simulink model "SingleTrackCANoe"  (R2021b)
settings: Solver=ode1  StartTime=0  StopTime=2  FixedStep=1.0000000000000000e-003  RelTol=1e-3
InitFcn:
  | sampleTime = str2double(get_param(bdroot, 'FixedStep'));
undefined symbols (not defined in the file or in its folder): AccPedalPos, BrakePedalPos, BrakeSwitch, DiscIntNeverNeededParam, DYNA4, EngSpd, IgnitionSwitch, InitialGear, InitialSpeed, IntendedEngTrq, LeftIndicator, MainBrakePress, MaxGear, MDL, MinGear, RefAcc, RefLane, RefLatPos, RefPath, RefPathCurv, RefSpd, RefSpdPreview, RefSpdRetrospect, RightIndicator, SteeringWheelAng, SteeringWheelTrq, UserDefinedRefValue, vm_const
libraries: UtilitiesLibrary x62, simulink x18, WheelSystemModules x14, LongitudinalControllerModules x13, LateralControllerModules x7, AnimationBusselectorModules x5, EnvironmentModules x5, BasicEngineControlModules x5, MiscellaneousControlModules x5, Animation3Modules x4, AuxiliariesModules x4, ReducedTireModules x4
(part 19 of 34)

== system SingleTrackCANoe/SimulationModel/Vehicle/Drivetrain/DrivetrainControlUnit/InputFromCTRL ==
  fromCTRL : Inport
  TDBusSelector : BusSelector  OutputSignals=CTRL.LongitudinalControl.TransmissionLoad[0_1],CTRL.LongitudinalControl.IntendedEngTrqActive[0;1],CTRL.LongitudinalControl.AccPedalPos[0_1],CTRL.LongitudinalControl.InitialGear[-4;20],CTRL.LongitudinalControl.MaxGear[-4;20],CTRL.LongitudinalControl.MinGear[-4;20],CTRL.LongitudinalControl.ShiftingProgramSelection[-],CTRL.LongitudinalControl.KickdownSwitch[0;1]
  __TDD__AccPedalPos[0_1] : Demux  Outputs=[1]
  __TDD__InitialGear[-4;20] : Demux  Outputs=[1]
  __TDD__IntendedEngTrqActive[0;1] : Demux  Outputs=[1]
  __TDD__KickdownSwitch[0;1] : Demux  Outputs=[1]
  __TDD__MaxGear[-4;20] : Demux  Outputs=[1]
  __TDD__MinGear[-4;20] : Demux  Outputs=[1]
  __TDD__ShiftingProgramSelection[-] : Demux  Outputs=[1]
  __TDD__TransmissionLoad[0_1] : Demux  Outputs=[1]
  TransmissionLoad[0_1]___UNIQUE_1 : Outport  Description=|  PortDimensions=[1]  VectorParamsAs1DForOutWhenUnconnected=off
      | <name>CTRL.LongitudinalControl.TransmissionLoad[0_1]</name>
      | <comment></comment>
  IntendedEngTrqActive[0;1]___UNIQUE_1 : Outport  Description=|  Port=2  PortDimensions=[1]  VectorParamsAs1DForOutWhenUnconnected=off
      | <name>CTRL.LongitudinalControl.IntendedEngTrqActive[0;1]</name>
      | <comment></comment>
  AccPedalPos[0_1]___UNIQUE_1 : Outport  Description=|  Port=3  PortDimensions=[1]  VectorParamsAs1DForOutWhenUnconnected=off
      | <name>CTRL.LongitudinalControl.AccPedalPos[0_1]</name>
      | <comment></comment>
  InitialGear[-4;20]___UNIQUE_1 : Outport  Description=|  Port=4  PortDimensions=[1]  VectorParamsAs1DForOutWhenUnconnected=off
      | <name>CTRL.LongitudinalControl.InitialGear[-4;20]</name>
      | <comment></comment>
  MaxGear[-4;20]___UNIQUE_1 : Outport  Description=|  Port=5  PortDimensions=[1]  VectorParamsAs1DForOutWhenUnconnected=off
      | <name>CTRL.LongitudinalControl.MaxGear[-4;20]</name>
      | <comment>Maximum gear</comment>
  MinGear[-4;20]___UNIQUE_1 : Outport  Description=|  Port=6  PortDimensions=[1]  VectorParamsAs1DForOutWhenUnconnected=off
      | <name>CTRL.LongitudinalControl.MinGear[-4;20]</name>
      | <comment>Minimum gear</comment>
  ShiftingProgramSelection[-]___UNIQUE_1 : Outport  Description=|  Port=7  PortDimensions=[1]  VectorParamsAs1DForOutWhenUnconnected=off
      | <name>CTRL.LongitudinalControl.ShiftingProgramSelection[-]</name>
      | <comment>Shifting program selection</comment>
  KickdownSwitch[0;1]___UNIQUE_1 : Outport  Description=|  Port=8  PortDimensions=[1]  VectorParamsAs1DForOutWhenUnconnected=off
      | <name>CTRL.LongitudinalControl.KickdownSwitch[0;1]</name>
      | <comment>Kickdown switch</comment>
  wires:
  __TDD__KickdownSwitch[0;1]/1 -> KickdownSwitch[0;1]___UNIQUE_1/1  "KickdownSwitch[0;1]"
  __TDD__ShiftingProgramSelection[-]/1 -> ShiftingProgramSelection[-]___UNIQUE_1/1  "ShiftingProgramSelection[-]"
  __TDD__MinGear[-4;20]/1 -> MinGear[-4;20]___UNIQUE_1/1  "MinGear[-4;20]"
  __TDD__MaxGear[-4;20]/1 -> MaxGear[-4;20]___UNIQUE_1/1  "MaxGear[-4;20]"
  __TDD__InitialGear[-4;20]/1 -> InitialGear[-4;20]___UNIQUE_1/1  "InitialGear[-4;20]"
  __TDD__AccPedalPos[0_1]/1 -> AccPedalPos[0_1]___UNIQUE_1/1  "AccPedalPos[0_1]"
  __TDD__IntendedEngTrqActive[0;1]/1 -> IntendedEngTrqActive[0;1]___UNIQUE_1/1  "IntendedEngTrqActive[0;1]"
  __TDD__TransmissionLoad[0_1]/1 -> TransmissionLoad[0_1]___UNIQUE_1/1  "TransmissionLoad[0_1]"
  TDBusSelector/8 -> __TDD__KickdownSwitch[0;1]/1  "<KickdownSwitch[0;1]>"
  TDBusSelector/7 -> __TDD__ShiftingProgramSelection[-]/1  "<ShiftingProgramSelection[-]>"
  TDBusSelector/6 -> __TDD__MinGear[-4;20]/1  "<MinGear[-4;20]>"
  TDBusSelector/5 -> __TDD__MaxGear[-4;20]/1  "<MaxGear[-4;20]>"
  TDBusSelector/4 -> __TDD__InitialGear[-4;20]/1  "<InitialGear[-4;20]>"
  TDBusSelector/3 -> __TDD__AccPedalPos[0_1]/1  "<AccPedalPos[0_1]>"
  TDBusSelector/2 -> __TDD__IntendedEngTrqActive[0;1]/1  "<IntendedEngTrqActive[0;1]>"
  TDBusSelector/1 -> __TDD__TransmissionLoad[0_1]/1  "<TransmissionLoad[0_1]>"
  fromCTRL/1 -> TDBusSelector/1

== system SingleTrackCANoe/SimulationModel/Vehicle/Drivetrain/DrivetrainControlUnit/InputFromDrivetrainPhysics ==
  fromDrivetrainPhysics : Inport
  TDBusSelector : BusSelector  OutputSignals=Transmission.Type[-],EngSpd[rad/s],Transmission.InSpd[rad/s],Transmission.OutSpd[rad/s],Transmission.NumFwdGears[-]
  __TDD__EngSpd[rad/s] : Demux  Outputs=[1]
  __TDD__InSpd[rad/s] : Demux  Outputs=[1]
  __TDD__NumFwdGears[-] : Demux  Outputs=[1]
  __TDD__OutSpd[rad/s] : Demux  Outputs=[1]
  __TDD__Type[-] : Demux  Outputs=1
  Type[-]___UNIQUE_1 : Outport  Description=|  VectorParamsAs1DForOutWhenUnconnected=off
      | <name>Transmission.Type[-]</name>
      | <comment></comment>
  EngSpd[rad/s] : Outport  Description=|  Port=2  PortDimensions=[1]  VectorParamsAs1DForOutWhenUnconnected=off
      | <name>EngSpd[rad/s]</name>
      | <comment>Engine speed</comment>
  InSpd[rad/s]___UNIQUE_1 : Outport  Description=|  Port=3  PortDimensions=[1]  VectorParamsAs1DForOutWhenUnconnected=off
      | <name>Transmission.InSpd[rad/s]</name>
      | <comment>Transmission input speed</comment>
  OutSpd[rad/s]___UNIQUE_1 : Outport  Description=|  Port=4  PortDimensions=[1]  VectorParamsAs1DForOutWhenUnconnected=off
      | <name>Transmission.OutSpd[rad/s]</name>
      | <comment>Transmission output speed</comment>
  NumFwdGears[-]___UNIQUE_1 : Outport  Description=|  Port=5  PortDimensions=[1]  VectorParamsAs1DForOutWhenUnconnected=off
      | <name>Transmission.NumFwdGears[-]</name>
      | <comment>Number of forward gears</comment>
  wires:
  __TDD__NumFwdGears[-]/1 -> NumFwdGears[-]___UNIQUE_1/1  "NumFwdGears[-]"
  __TDD__OutSpd[rad/s]/1 -> OutSpd[rad/s]___UNIQUE_1/1  "OutSpd[rad/s]"
  __TDD__InSpd[rad/s]/1 -> InSpd[rad/s]___UNIQUE_1/1  "InSpd[rad/s]"
  __TDD__EngSpd[rad/s]/1 -> EngSpd[rad/s]/1  "EngSpd[rad/s]"
  __TDD__Type[-]/1 -> Type[-]___UNIQUE_1/1  "Type[-]"
  TDBusSelector/5 -> __TDD__NumFwdGears[-]/1  "<NumFwdGears[-]>"
  TDBusSelector/4 -> __TDD__OutSpd[rad/s]/1  "<OutSpd[rad/s]>"
  TDBusSelector/3 -> __TDD__InSpd[rad/s]/1  "<InSpd[rad/s]>"
  TDBusSelector/2 -> __TDD__EngSpd[rad/s]/1  "<EngSpd[rad/s]>"
  TDBusSelector/1 -> __TDD__Type[-]/1  "<Type[-]>"
  fromDrivetrainPhysics/1 -> TDBusSelector/1

== system SingleTrackCANoe/SimulationModel/Vehicle/Drivetrain/DrivetrainControlUnit/TransmissionControlUnit ==
  AccPedalPos[0_1] : Inport  Description=Accelerator pedal position
  EngSpd[rad/s] : Inport  Description=Engine speed  Port=2
  TransmissionInSpd[rad/s] : Inport  Description=Transmission input speed  Port=3
  TransmissionOutSpd[rad/s] : Inport  Description=Transmission output speed  Port=4
  NumFwdGears[-] : Inport  Description=Number of forward gears  Port=5
  InitialGear[-4;20] : Inport  Description=Accelerator pedal position  Port=6
  MaxGear[-4;20] : Inport  Description=Maximum gear  Port=7
  MinGear[-4;20] : Inport  Description=Minimum gear  Port=8
  ShiftingProgramSelection[-] : Inport  Description=Shifting program selection  Port=9
  KickdownSwitch[0;1] : Inport  Description=Kick-down switch  Port=10
  Enable : EnablePort  StatesWhenEnabling=reset
  TransmissionControlUnit : TransmissionControlModules/TransmissionControlUnit  DATA_NODE=MDL.Vehicle.Drivetrain.DrivetrainControlUnit.TransmissionControlUnit  GearChangeMinTime=MDL.Vehicle.Drivetrain.DrivetrainControlUnit.TransmissionControlUnit.GearChangeMinTime  GearChangeDelay=MDL.Vehicle.Drivetrain.DrivetrainControlUnit.TransmissionControlUnit.GearChangeDelay  EngSpdFilterTimeConst=MDL.Vehicle.Drivetrain.DrivetrainControlUnit.TransmissionControlUnit.EngSpdFilterTimeConst  LockUpClutchOpenTime=MDL.Vehicle.Drivetrain.DrivetrainControlUnit.TransmissionControlUnit.LockUpClutch.OpenTime  LockUpClutchCloseTime=MDL.Vehicle.Drivetrain.DrivetrainControlUnit.TransmissionControlUnit.LockUpClutch.CloseTime  ThresKickdownOpenControlled=MDL.Vehicle.Drivetrain.DrivetrainControlUnit.TransmissionControlUnit.LockUpClutch.KickDownMode.OpenToControlledSpdCurve  ThresKickdownControlledOpen=MDL.Vehicle.Drivetrain.DrivetrainControlUnit.TransmissionControlUnit.LockUpClutch.KickDownMode.ControlledToOpenSpdCurve  ThresKickdownClosedControlled=MDL.Vehicle.Drivetrain.DrivetrainControlUnit.TransmissionControlUnit.LockUpClutch.KickDownMode.ClosedToControlledSpdCurve  ThresKickdownControlledClosed=MDL.Vehicle.Drivetrain.DrivetrainControlUnit.TransmissionControlUnit.LockUpClutch.KickDownMode.ControlledToClosedSpdCurve  ThresOpenControlled=MDL.Vehicle.Drivetrain.DrivetrainControlUnit.TransmissionControlUnit.LockUpClutch.RegularMode.OpenToControlledSpdMap3D  ThresControlledOpen=MDL.Vehicle.Drivetrain.DrivetrainControlUnit.TransmissionControlUnit.LockUpClutch.RegularMode.ControlledToOpenSpdMap3D  ThresClosedControlled=MDL.Vehicle.Drivetrain.DrivetrainControlUnit.TransmissionControlUnit.LockUpClutch.RegularMode.ClosedToControlledSpdMap3D  ThresControlledClosed=MDL.Vehicle.Drivetrain.DrivetrainControlUnit.TransmissionControlUnit.LockUpClutch.RegularMode.ControlledToClosedSpdMap3D  OpenClutchDelay=MDL.Vehicle.Drivetrain.DrivetrainControlUnit.TransmissionControlUnit.ManualClutch.OpenClutchDelay  ClutchPedalCorrectFac=MDL.Vehicle.Drivetrain.DrivetrainControlUnit.TransmissionControlUnit.ManualClutch.ClutchPedalCorrectFacCurve  ClutchOpenTime=MDL.Vehicle.Drivetrain.DrivetrainControlUnit.TransmissionControlUnit.ManualClutch.OpenTime  OpenClutchDuration=MDL.Vehicle.Drivetrain.DrivetrainControlUnit.TransmissionControlUnit.ManualClutch.OpenClutchDuration  ClutchCloseTime=MDL.Vehicle.Drivetrain.DrivetrainControlUnit.TransmissionControlUnit.ManualClutch.CloseTime  LowerGearLimit=MDL.Vehicle.Drivetrain.DrivetrainControlUnit.TransmissionControlUnit.ShiftingProgram.DirectShifting.LowerGearLimit  TransmissionOutSpdThres=MDL.Vehicle.Drivetrain.DrivetrainControlUnit.TransmissionControlUnit.ShiftingProgram.DirectShifting.Spd  KickdownShiftUp=MDL.Vehicle.Drivetrain.DrivetrainControlUnit.TransmissionControlUnit.ShiftingProgram.KickDownMode.UpshiftSpdCurve  KickdownShiftDown=MDL.Vehicle.Drivetrain.DrivetrainControlUnit.TransmissionControlUnit.ShiftingProgram.KickDownMode.DownshiftSpdCurve  ShiftUp=MDL.Vehicle.Drivetrain.DrivetrainControlUnit.TransmissionControlUnit.ShiftingProgram.RegularMode.UpshiftSpdMap3D  ShiftDown=MDL.Vehicle.Drivetrain.DrivetrainControlUnit.TransmissionControlUnit.ShiftingProgram.RegularMode.DownshiftSpdMap3D  SlipCtrlClutchSlip=MDL.Vehicle.Drivetrain.DrivetrainControlUnit.TransmissionControlUnit.SlipController.ClutchIntendedSlipMap3D  SlipCtrlProportionalGain=MDL.Vehicle.Drivetrain.DrivetrainControlUnit.TransmissionControlUnit.SlipController.ProportionalGain  SlipCtrlIntegralGain=MDL.Vehicle.Drivetrain.DrivetrainControlUnit.TransmissionControlUnit.SlipController.IntegralGain  SlipCtrlTimeConst=MDL.Vehicle.Drivetrain.DrivetrainControlUnit.TransmissionControlUnit.SlipController.TimeConst  TractionCtrlIntTrq=MDL.Vehicle.Drivetrain.DrivetrainControlUnit.TransmissionControlUnit.TractionController.RefEngTrq  ASREndClutchPos=MDL.Vehicle.Drivetrain.DrivetrainControlUnit.TransmissionControlUnit.TractionController.ASREndClutchPos
  Gear[-4;20] : Outport  Description=Gear  OutputWhenDisabled=reset  InitialOutput=0  VectorParamsAs1DForOutWhenUnconnected=off
  LockUpClutchPos[0_1] : Outport  Description=Lock-up clutch position  Port=2  OutputWhenDisabled=reset  InitialOutput=0  VectorParamsAs1DForOutWhenUnconnected=off
  AutomatedManualClutchPos[0_1] : Outport  Description=Clutch position for manual shifting  Port=3  OutputWhenDisabled=reset  InitialOutput=0  VectorParamsAs1DForOutWhenUnconnected=off
  GearTarget[-4;20] : Outport  Description=ASR torque  Port=4  OutputWhenDisabled=reset  InitialOutput=0  VectorParamsAs1DForOutWhenUnconnected=off
  ASRRequestSwitch[0;2] : Outport  Description=Switch indicating if no ASR (0), slow ASR (1), or fast ASR (2) is requested  Port=5  OutputWhenDisabled=reset  InitialOutput=0  VectorParamsAs1DForOutWhenUnconnected=off
  ASRTrq[Nm] : Outport  Description=ASR torque  Port=6  OutputWhenDisabled=reset  InitialOutput=0  VectorParamsAs1DForOutWhenUnconnected=off
  wires:
  InitialGear[-4;20]/1 -> TransmissionControlUnit/6
  NumFwdGears[-]/1 -> TransmissionControlUnit/5
  TransmissionOutSpd[rad/s]/1 -> TransmissionControlUnit/4
  EngSpd[rad/s]/1 -> TransmissionControlUnit/2
  AccPedalPos[0_1]/1 -> TransmissionControlUnit/1
  TransmissionInSpd[rad/s]/1 -> TransmissionControlUnit/3
  KickdownSwitch[0;1]/1 -> TransmissionControlUnit/10
  TransmissionControlUnit/6 -> GearTarget[-4;20]/1
  ShiftingProgramSelection[-]/1 -> TransmissionControlUnit/9
  MinGear[-4;20]/1 -> TransmissionControlUnit/8
  MaxGear[-4;20]/1 -> TransmissionControlUnit/7
  TransmissionControlUnit/1 -> Gear[-4;20]/1
  TransmissionControlUnit/2 -> LockUpClutchPos[0_1]/1
  TransmissionControlUnit/3 -> AutomatedManualClutchPos[0_1]/1
  TransmissionControlUnit/4 -> ASRRequestSwitch[0;2]/1
  TransmissionControlUnit/5 -> ASRTrq[Nm]/1

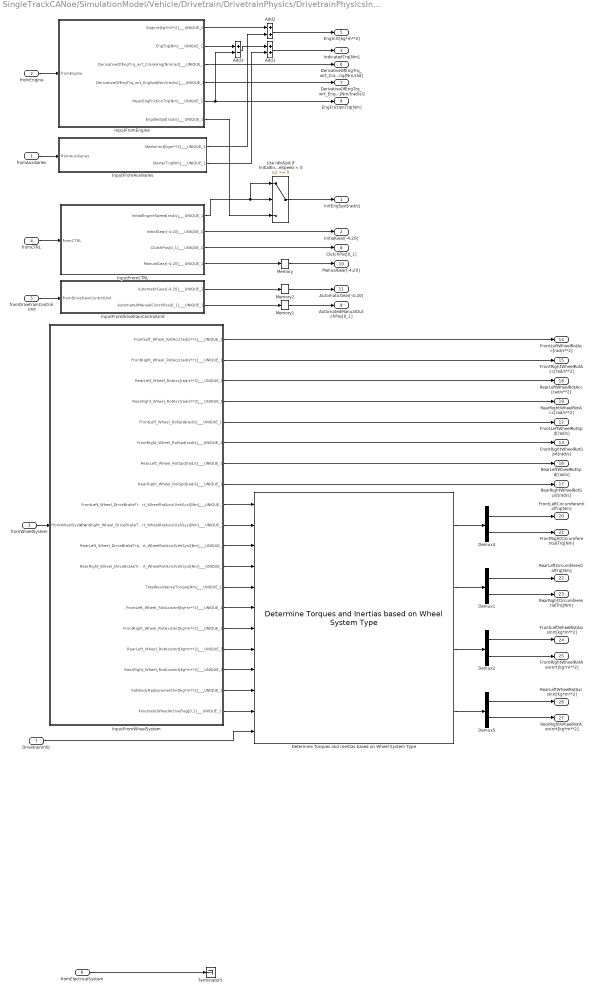
== system SingleTrackCANoe/SimulationModel/Vehicle/Drivetrain/DrivetrainPhysics/DrivetrainPhysicsInputs ==
  fromAuxiliaries : Inport
  fromEngine : Inport  Port=2
  fromWheelSystem : Inport  Port=3
  fromCTRL : Inport  Port=4
  fromDrivetrainControlUnit : Inport  Port=5
  fromElectricalSystem : Inport  Port=6
  DrivetrainInfo : Inport  Port=7
  Add1 : Sum
  Add2 : Sum
  Add3 : Sum  Inputs=+-
  Demux{1..2,4..5} (4 alike) : Demux  Outputs=2
  Determine Torques and Inertias based on Wheel System Type : DrivetrainModules/Determine Torques and Inertias based on Wheel System Type  SystemSampleTime=-1  VariantActivationTime=update diagram  Latency=0  AutoFrameSizeCalculation=off
  InputFromAuxiliaries : Subsystem  Tag=TESIS DYNAware Interface Block  mask{NeedsUpdate=off, SignalInfo=|}
      mask SignalInfo=|
      | {
      |   "Version": "4.6",
      |   "MuxedOutputBusName": "output",
      |   "MuxedInputBusName": "fromAuxiliaries",
      |   "MuxedInputSelected": true,
      |   "MuxedOutputSelected": false,
      |   "SignalData": [
      |     {
      |       "initialValue": "0.0",
      |       "name": "StarterInrt[kgm**2]",
      |       "comment": "",
      |       "minString": "",
      |       "maxString": "",
      |       "width": 1,
      |       "dataType": 0,
      |       "signalType": 0,
      |       "createSignal": false,
      |       "outputName": "StarterInrt[kgm**2]",
      |       "generateSignalAccessBlock": false,
      |       "accessId": "$(parentId).$(blockName).$(outputName)"
      |     },
      |     {
      |       "initialValue": "0.0",
      |       "name": "StarterTrq[Nm]",
      |       "comment": "",
      |       "minString": "",
      |       "maxString": "",
      |       "width": 1,
      |       "dataType": 0,
      |       "signalType": 0,
      |       "createSignal": false,
      |       "outputName": "StarterTrq[Nm]",
      |       "generateSignalAccessBlock": false,
      |       "accessId": "$(parentId).$(blockName).$(outputName)"
      |     }
      |   ]
      | }
      mask prompts: NeedsUpdate "Specify, if subsystem content needs to be updated"; SignalInfo "Signal Info (json)"
      mask help: DYNA4 Interface Block Version 4.6
      mask init:
      | blockName = get_param(gcbh, 'Name');
      | parentId = DYNA4.ModelHandling.AccessID.getFromHierarchy(gcbh);
      | TD.InterfaceBlock.ModelCallbacks.GenerateContent(gcb);
      settings: DeleteFcn=TD.InterfaceBlock.ModelCallbacks.CloseGUI( gcbh );  NameChangeFcn=TD.InterfaceBlock.ModelCallbacks.BlockRenamedHandler(gcbh);  OpenFcn=TD.InterfaceBlock.ModelCallbacks.OpenGUI( gcbh );  CloseFcn=TD.InterfaceBlock.ModelCallbacks.CloseGUI( gcbh );
      mask Display:
      | image('InterfaceBlock.png','center');
      | port_label('input',1, 'fromAuxiliaries');
      | port_label('output',1, 'StarterInrt[kgm**2]');
      | port_label('output',2, 'StarterTrq[Nm]');
  InputFromCTRL : Subsystem  Tag=TESIS DYNAware Interface Block  mask{NeedsUpdate=off, SignalInfo=|}
      mask SignalInfo=|
      | {
      |   "Version": "4.6",
      |   "MuxedOutputBusName": "output",
      |   "MuxedInputBusName": "fromCTRL",
      |   "MuxedInputSelected": true,
      |   "MuxedOutputSelected": false,
      |   "SignalData": [
      |     {
      |       "initialValue": "0.0",
      |       "name": "CTRL.LongitudinalControl.InitialEngineSpeed[rad/s]",
      |       "comment": "",
      |       "minString": "",
      |       "maxString": "",
      |       "width": 1,
      |       "dataType": 0,
      |       "signalType": 0,
      |       "createSignal": false,
      |       "outputName": "InitialEngineSpeed[rad/s]",
      |       "generateSignalAccessBlock": false,
      |       "accessId": "$(parentId).$(blockName).$(outputName)"
      |     },
      |     {
      |       "initialValue": "0.0",
      |       "name": "CTRL.LongitudinalControl.InitialGear[-4;20]",
      |       "comment": "",
      |       "minString": "",
      |       "maxString": "",
      |       "width": 1,
      |       "dataType": 0,
      |       "signalType": 0,
      |       "createSignal": false,
      |       "outputName": "InitialGear[-4;20]",
      |       "generateSignalAccessBlock": false,
      |       "accessId": "$(parentId).$(blockName).$(outputName)"
      |     },
      |     {
      |       "initialValue": "0.0",
      |       "name": "CTRL.LongitudinalControl.ClutchPos[0_1]",
      |       "comment": "",
      |       "minString": "",
      |       "maxString": "",
      |       "width": 1,
      |       "dataType": 0,
      |       "signalType": 0,
      |       "createSignal": false,
      |       "outputName": "ClutchPos[0_1]",
      |       "generateSignalAccessBlock": false,
      |       "accessId": "$(parentId).$(blockName).$(outputName)"
      |     },
      |     {
      |       "initialValue": "0.0",
      |       "name": "CTRL.LongitudinalControl.ManualGear[-4;20]",
      |       "comment": "",
      |       "minString": "",
      |       "maxString": "",
      |       "width": 1,
      |       "dataType": 0,
      |       "signalType": 0,
      |       "createSignal": false,
      |       "outputName": "ManualGear[-4;20]",
      |       "generateSignalAccessBlock": false,
      |       "accessId": "$(parentId).$(blockName).$(outputName)"
      |     }
      |   ]
      | }
      mask prompts: NeedsUpdate "Specify, if subsystem content needs to be updated"; SignalInfo "Signal Info (json)"
      mask help: DYNA4 Interface Block Version 4.6
      mask init:
      | blockName = get_param(gcbh, 'Name');
      | parentId = DYNA4.ModelHandling.AccessID.getFromHierarchy(gcbh);
      | TD.InterfaceBlock.ModelCallbacks.GenerateContent(gcb);
      settings: DeleteFcn=TD.InterfaceBlock.ModelCallbacks.CloseGUI( gcbh );  NameChangeFcn=TD.InterfaceBlock.ModelCallbacks.BlockRenamedHandler(gcbh);  OpenFcn=TD.InterfaceBlock.ModelCallbacks.OpenGUI( gcbh );  CloseFcn=TD.InterfaceBlock.ModelCallbacks.CloseGUI( gcbh );
      mask Display:
      | image('InterfaceBlock.png','center');
      | port_label('input',1, 'fromCTRL');
      | port_label('output',1, 'InitialEngineSpeed[rad/s]');
      | port_label('output',2, 'InitialGear[-4;20]');
      | port_label('output',3, 'ClutchPos[0_1]');
      | port_label('output',4, 'ManualGear[-4;20]');
  InputFromDrivetrainControlUnit : Subsystem  Tag=TESIS DYNAware Interface Block  mask{NeedsUpdate=off, SignalInfo=|}
      mask SignalInfo=|
      | {
      |   "Version": "4.6",
      |   "MuxedOutputBusName": "output",
      |   "MuxedInputBusName": "fromDrivetrainControlUnit",
      |   "MuxedInputSelected": true,
      |   "MuxedOutputSelected": false,
      |   "SignalData": [
      |     {
      |       "initialValue": "0.0",
      |       "name": "TransmissionControlUnit.Gear[-4;20]",
      |       "comment": "",
      |       "minString": "",
      |       "maxString": "",
      |       "width": 1,
      |       "dataType": 0,
      |       "signalType": 0,
      |       "createSignal": false,
      |       "outputName": "AutomaticGear[-4;20]",
      |       "generateSignalAccessBlock": false,
      |       "accessId": "$(parentId).$(blockName).$(outputName)"
      |     },
      |     {
      |       "initialValue": "0.0",
      |       "name": "TransmissionControlUnit.AutomatedManualClutchPos[0_1]",
      |       "comment": "",
      |       "minString": "",
      |       "maxString": "",
      |       "width": 1,
      |       "dataType": 0,
      |       "signalType": 0,
      |       "createSignal": false,
      |       "outputName": "AutomatedManualClutchPos[0_1]",
      |       "generateSignalAccessBlock": false,
      |       "accessId": "$(parentId).$(blockName).$(outputName)"
      |     }
      |   ]
      | }
      mask prompts: NeedsUpdate "Specify, if subsystem content needs to be updated"; SignalInfo "Signal Info (json)"
      mask help: DYNA4 Interface Block Version 4.6
      mask init:
      | blockName = get_param(gcbh, 'Name');
      | parentId = DYNA4.ModelHandling.AccessID.getFromHierarchy(gcbh);
      | TD.InterfaceBlock.ModelCallbacks.GenerateContent(gcb);
      settings: DeleteFcn=TD.InterfaceBlock.ModelCallbacks.CloseGUI( gcbh );  NameChangeFcn=TD.InterfaceBlock.ModelCallbacks.BlockRenamedHandler(gcbh);  OpenFcn=TD.InterfaceBlock.ModelCallbacks.OpenGUI( gcbh );  CloseFcn=TD.InterfaceBlock.ModelCallbacks.CloseGUI( gcbh );
      mask Display:
      | image('InterfaceBlock.png','center');
      | port_label('input',1, 'fromDrivetrainControlUnit');
      | port_label('output',1, 'AutomaticGear[-4;20]');
      | port_label('output',2, 'AutomatedManualClutchPos[0_1]');
  InputFromEngine : Subsystem  Tag=TESIS DYNAware Interface Block  mask{NeedsUpdate=off, SignalInfo=|}
      mask SignalInfo=|
      | {
      |   "Version": "4.6",
      |   "MuxedOutputBusName": "Drivetrain",
      |   "MuxedInputBusName": "fromEngine",
      |   "MuxedInputSelected": true,
      |   "MuxedOutputSelected": false,
      |   "SignalData": [
      |     {
      |       "initialValue": "0.0",
      |       "name": "EnginePhysics.Mechanics.EngInrt[kg*m**2]",
      |       "comment": "",
      |       "minString": "",
      |       "maxString": "",
      |       "width": 1,
      |       "dataType": 0,
      |       "signalType": 0,
      |       "createSignal": false,
      |       "outputName": "EngInrt[kg*m**2]",
      |       "generateSignalAccessBlock": false,
      |       "accessId": "$(parentId).$(blockName).$(outputName)"
      |     },
      |     {
      |       "initialValue": "0.0",
      |       "name": "EnginePhysics.Mechanics.EngTrq[Nm]",
      |       "comment": "",
      |       "minString": "",
      |       "maxString": "",
      |       "width": 1,
      |       "dataType": 0,
      |       "signalType": 0,
      |       "createSignal": false,
      |       "outputName": "EngTrq[Nm]",
      |       "generateSignalAccessBlock": false,
      |       "accessId": "$(parentId).$(blockName).$(outputName)"
      |     },
      |     {
      |       "initialValue": "0.0",
      |       "name": "EnginePhysics.Mechanics.DerivativeOfEngTrq_wrt_CrankAng[Nm/rad]",
      |       "comment": "",
      |       "minString": "",
      |       "maxString": "",
      |       "width": 1,
      |       "dataType": 0,
      |       "signalType": 0,
      |       "createSignal": false,
      |       "outputName": "DerivativeOfEngTrq_wrt_CrankAng[Nm/rad]",
      |       "generateSignalAccessBlock": false,
      |       "accessId": "$(parentId).$(blockName).$(outputName)"
      |     },
      |     {
      |       "initialValue": "0.0",
      |       "name": "EnginePhysics.Mechanics.DerivativeOfEngTrq_wrt_EngSpd[Nm/(rad/s)]",
      |       "comment": "",
      |       "minString": "",
      |       "maxString": "",
      |       "width": 1,
      |       "dataType": 0,
      |       "signalType": 0,
      |       "createSignal": false,
      |       "outputName": "DerivativeOfEngTrq_wrt_EngSpd[Nm/(rad/s)]",
      |       "generateSignalAccessBlock": false,
      |       "accessId": "$(parentId).$(blockName).$(outputName)"
      |     },
      |     {
      |       "initialValue": "0.0",
      |       "name": "EnginePhysics.Mechanics.MeanEngFrictionTrq[Nm]",
      |       "comment": "",
      |       "minString": "",
      |       "maxString": "",
      |       "width": 1,
      |       "dataType": 0,
      |       "signalType": 0,
      |       "createSignal": false,
      |       "outputName": "MeanEngFrictionTrq[Nm]",
      |       "generateSignalAccessBlock": false,
      |       "accessId": "$(parentId).$(blockName).$(outputName)"
      |     },
      |     {
      |       "initialValue": "0.0",
      |       "name": "EngineControlUnit.EngIdleSpd[rad/s]",
      |       "comment": "",
      |       "minString": "",
      |       "maxString": "",
      |       "width": 1,
      |       "dataType": 0,
      |       "signalType": 0,
      |       "createSignal": false,
      |       "outputName": "EngIdleSpd[rad/s]",
      |       "generateSignalAccessBlock": false,
      |       "accessId": "$(parentId).$(blockName).$(outputName)"
      |     }
      |   ]
      | }
      mask prompts: NeedsUpdate "Specify, if subsystem content needs to be updated"; SignalInfo "Signal Info (json)"
      mask help: DYNA4 Interface Block Version 4.6
      mask init:
      | blockName = get_param(gcbh, 'Name');
      | parentId = DYNA4.ModelHandling.AccessID.getFromHierarchy(gcbh);
      | TD.InterfaceBlock.ModelCallbacks.GenerateContent(gcb);
      settings: DeleteFcn=TD.InterfaceBlock.ModelCallbacks.CloseGUI( gcbh );  NameChangeFcn=TD.InterfaceBlock.ModelCallbacks.BlockRenamedHandler(gcbh);  OpenFcn=TD.InterfaceBlock.ModelCallbacks.OpenGUI( gcbh );  CloseFcn=TD.InterfaceBlock.ModelCallbacks.CloseGUI( gcbh );
      mask Display:
      | image('InterfaceBlock.png','center');
      | port_label('input',1, 'fromEngine');
      | port_label('output',1, 'EngInrt[kg*m**2]');
      | port_label('output',2, 'EngTrq[Nm]');
      | port_label('output',3, 'DerivativeOfEngTrq_wrt_CrankAng[Nm/rad]');
      | port_label('output',4, 'DerivativeOfEngTrq_wrt_EngSpd[Nm/(rad/s)]');
      | port_label('output',5, 'MeanEngFrictionTrq[Nm]');
      | port_label('output',6, 'EngIdleSpd[rad/s]');
  InputFromWheelSystem : Subsystem  Tag=TESIS DYNAware Interface Block  mask{NeedsUpdate=off, SignalInfo=|}
      mask SignalInfo=|
      | {
      |   "Version": "4.6",
      |   "MuxedOutputBusName": "output",
      |   "MuxedInputBusName": "fromWheelSystem",
      |   "MuxedInputSelected": true,
      |   "MuxedOutputSelected": false,
      |   "SignalData": [
      |     {
      |       "initialValue": "0.0",
      |       "name": "FrontLeft.Wheel.RotAcc[rad/s**2]",
      |       "comment": "",
      |       "minString": "",
      |       "maxString": "",
      |       "width": -1,
      |       "dataType": 0,
      |       "signalType": 0,
      |       "createSignal": false,
      |       "outputName": "FrontLeft_Wheel_RotAcc[rad/s**2]",
      |       "generateSignalAccessBlock": false,
      |       "accessId": "$(parentId).$(blockName).$(outputName)"
      |     },
      |     {
      |       "initialValue": "0.0",
      |       "name": "FrontRight.Wheel.RotAcc[rad/s**2]",
      |       "comment": "",
      |       "minString": "",
      |       "maxString": "",
      |       "width": -1,
      |       "dataType": 0,
      |       "signalType": 0,
      |       "createSignal": false,
      |       "outputName": "FrontRight_Wheel_RotAcc[rad/s**2]",
      |       "generateSignalAccessBlock": false,
      |       "accessId": "$(parentId).$(blockName).$(outputName)"
      |     },
      |     {
      |       "initialValue": "0.0",
      |       "name": "RearLeft.Wheel.RotAcc[rad/s**2]",
      |       "comment": "",
      |       "minString": "",
      |       "maxString": "",
      |       "width": -1,
      |       "dataType": 0,
      |       "signalType": 0,
      |       "createSignal": false,
      |       "outputName": "RearLeft_Wheel_RotAcc[rad/s**2]",
      |       "generateSignalAccessBlock": false,
      |       "accessId": "$(parentId).$(blockName).$(outputName)"
      |     },
      |     {
      |       "initialValue": "0.0",
      |       "name": "RearRight.Wheel.RotAcc[rad/s**2]",
      |       "comment": "",
      |       "minString": "",
      |       "maxString": "",
      |       "width": -1,
      |       "dataType": 0,
      |       "signalType": 0,
      |       "createSignal": false,
      |       "outputName": "RearRight_Wheel_RotAcc[rad/s**2]",
      |       "generateSignalAccessBlock": false,
      |       "accessId": "$(parentId).$(blockName).$(outputName)"
      |     },
      |     {
      |       "initialValue": "0.0",
      |       "name": "FrontLeft.Wheel.RotSpd[rad/s]",
      |       "comment": "",
      |       "minString": "",
      |       "maxString": "",
      |       "width": 1,
      |       "dataType": 0,
      |       "signalType": 0,
      |       "createSignal": false,
      |       "outputName": "FrontLeft_Wheel_RotSpd[rad/s]",
      |       "generateSignalAccessBlock": false,
      |       "accessId": "$(parentId).$(blockName).$(outputName)"
      |     },
      |     {
      |       "initialValue": "0.0",
      |       "name": "FrontRight.Wheel.RotSpd[rad/s]",
      |       "comment": "",
      |       "minString": "",
      |       "maxString": "",
      |       "width": 1,
      |       "dataType": 0,
      |       "signalType": 0,
      |       "createSignal": false,
      |       "outputName": "FrontRight_Wheel_RotSpd[rad/s]",
      |       "generateSignalAccessBlock": false,
      |       "accessId": "$(parentId).$(blockName).$(outputName)"
      |     },
      |     {
      |       "initialValue": "0.0",
      |       "name": "RearLeft.Wheel.RotSpd[rad/s]",
      |       "comment": "",
      |       "minString": "",
      |       "maxString": "",
      |       "width": 1,
      |       "dataType": 0,
      |       "signalType": 0,
      |       "createSignal": false,
      |       "outputName": "RearLeft_Wheel_RotSpd[rad/s]",
      |       "generateSignalAccessBlock": false,
      |       "accessId": "$(parentId).$(blockName).$(outputName)"
      |     },
      |     {
      |       "initialValue": "0.0",
      |       "name": "RearRight.Wheel.RotSpd[rad/s]",
      |       "comment": "",
      |       "minString": "",
      |       "maxString": "",
      |       "width": 1,
      |       "dataType": 0,
      |       "signalType": 0,
      |       "createSignal": false,
      |       "outputName": "RearRight_Wheel_RotSpd[rad/s]",
      |       "generateSignalAccessBlock": false,
      |       "accessId": "$(parentId).$(blockName).$(outputName)"
      |     },
      |     {
      |       "initialValue": "0.0",
      |       "name": "FrontLeft.Wheel.DriveBrakeTrq_wrt_WheelRotAxis(VehSys)[Nm]",
      |       "comment": "",
      |       "minString": "",
      |       "maxString": "",
      |       "width": 3,
      |       "dataType": 0,
      |       "signalType": 0,
      |       "createSignal": false,
      |       "outputName": "FrontLeft_Wheel_DriveBrakeTrq_wrt_WheelRotAxis(VehSys)[Nm]",
      |       "generateSignalAccessBlock": false,
      |       "accessId": "$(parentId).$(blockName).$(outputName)"
      |     },
      |     {
      |       "initialValue": "0.0",
      |       "name": "FrontRight.Wheel.DriveBrakeTrq_wrt_WheelRotAxis(VehSys)[Nm]",
      |       "comment": "",
      |       "minString": "",
      |       "maxString": "",
      |       "width": 3,
      |       "dataType": 0,
      |       "signalType": 0,
      |       "createSignal": false,
      |       "outputName": "FrontRight_Wheel_DriveBrakeTrq_wrt_WheelRotAxis(VehSys)[Nm]",
      |       "generateSignalAccessBlock": false,
      |       "accessId": "$(parentId).$(blockName).$(outputName)"
      |     },
      |     {
      |       "initialValue": "0.0",
      |       "name": "RearLeft.Wheel.DriveBrakeTrq_wrt_WheelRotAxis(VehSys)[Nm]",
      |       "comment": "",
      |       "minString": "",
      |       "maxString": "",
      |       "width": 3,
      |       "dataType": 0,
      |       "signalType": 0,
      |       "createSignal": false,
      |       "outputName": "RearLeft_Wheel_DriveBrakeTrq_wrt_WheelRotAxis(VehSys)[Nm]",
      |       "generateSignalAccessBlock": false,
      |       "accessId": "$(parentId).$(blockName).$(outputName)"
      |     },
      |     {
      |       "initialValue": "0.0",
      |       "name": "RearRight.Wheel.DriveBrakeTrq_wrt_WheelRotAxis(VehSys)[Nm]",
      |       "comment": "",
      |       "minString": "",
      |       "maxString": "",
      |       "width": 3,
      |       "dataType": 0,
      |       "signalType": 0,
      |       "createSignal": false,
      |       "outputName": "RearRight_Wheel_DriveBrakeTrq_wrt_WheelRotAxis(VehSys)[Nm]",
      |       "generateSignalAccessBlock": false,
      |       "accessId": "$(parentId).$(blockName).$(outputName)"
      |     },
      |     {
      |       "initialValue": "0.0",
      |       "name": "FrontLeft.Wheel.TotalResistanceTorque[Nm]",
      |       "comment": "",
      |       "minString": "",
      |       "maxString": "",
      |       "width": 1,
      |       "dataType": 0,
      |       "signalType": 0,
      |       "createSignal": false,
      |       "outputName": "TotalResistanceTorque[Nm]",
      |       "generateSignalAccessBlock": false,
      |       "accessId": "$(parentId).$(blockName).$(outputName)"
      |     },
      |     {
      |       "initialValue": "0.0",
      |       "name": "FrontLeft.Wheel.RotAxisInrt[kg*m**2]",
      |       "comment": "",
      |       "minString": "",
      |       "maxString": "",
      |       "width": 1,
      |       "dataType": 0,
      |       "signalType": 0,
      |       "createSignal": false,
      |       "outputName": "FrontLeft_Wheel_RotAxisInrt[kg*m**2]",
      |       "generateSignalAccessBlock": false,
      |       "accessId": "$(parentId).$(blockName).$(outputName)"
      |     },
      |     {
      |       "initialValue": "0.0",
      |       "name": "FrontRight.Wheel.RotAxisInrt[kg*m**2]",
      |       "comment": "",
      |       "minString": "",
      |       "maxString": "",
      |       "width": 1,
      |       "dataType": 0,
      |       "signalType": 0,
      |       "createSignal": false,
      |       "outputName": "FrontRight_Wheel_RotAxisInrt[kg*m**2]",
      |       "generateSignalAccessBlock": false,
      |       "accessId": "$(parentId).$(blockName).$(outputName)"
      |     },
      |     {
      |       "initialValue": "0.0",
      |       "name": "RearLeft.Wheel.RotAxisInrt[kg*m**2]",
      |       "comment": "",
      |       "minString": "",
      |       "maxString": "",
      |       "width": 1,
      |       "dataType": 0,
      |       "signalType": 0,
      |       "createSignal": false,
      |       "outputName": "RearLeft_Wheel_RotAxisInrt[kg*m**2]",
      |       "generateSignalAccessBlock": false,
      |       "accessId": "$(parentId).$(blockName).$(outputName)"
      |     },
      |     {
      |       "initialValue": "0.0",
      |       "name": "RearRight.Wheel.RotAxisInrt[kg*m**2]",
      |       "comment": "",
      |       "minString": "",
      |       "maxString": "",
      |       "width": 1,
      |       "dataType": 0,
      |       "signalType": 0,
      |       "createSignal": false,
      |       "outputName": "RearRight_Wheel_RotAxisInrt[kg*m**2]",
      |       "generateSignalAccessBlock": false,
      |       "accessId": "$(parentId).$(blockName).$(outputName)"
      |     },
      |     {
      |       "initialValue": "0.0",
      |       "name": "FrontLeft.Wheel.VehBodyReplacementInrt[kg*m**2]",
      |       "comment": "",
      |       "minString": "",
      |       "maxString": "",
      |       "width": 1,
      |       "dataType": 0,
      |       "signalType": 0,
      |       "createSignal": false,
      |       "outputName": "VehBodyReplacementInrt[kg*m**2]",
      |       "generateSignalAccessBlock": false,
      |       "accessId": "$(parentId).$(blockName).$(outputName)"
      |     },
      |     {
      |       "initialValue": "0.0",
      |       "name": "FrontLeft.Wheel.KinematicWheelActiveFlag[0;1]",
      |       "comment": "",
      |       "minString": "",
      |       "maxString": "",
      |       "width": 1,
      |       "dataType": 0,
      |       "signalType": 0,
      |       "createSignal": false,
      |       "outputName": "KinematicWheelActiveFlag[0;1]",
      |       "generateSignalAccessBlock": false,
      |       "accessId": "$(parentId).$(blockName).$(outputName)"
      |     }
      |   ]
      | }
      mask prompts: NeedsUpdate "Specify, if subsystem content needs to be updated"; SignalInfo "Signal Info (json)"
      mask help: DYNA4 Interface Block Version 4.6
      mask init:
      | blockName = get_param(gcbh, 'Name');
      | parentId = DYNA4.ModelHandling.AccessID.getFromHierarchy(gcbh);
      | TD.InterfaceBlock.ModelCallbacks.GenerateContent(gcb);
      settings: DeleteFcn=TD.InterfaceBlock.ModelCallbacks.CloseGUI( gcbh );  NameChangeFcn=TD.InterfaceBlock.ModelCallbacks.BlockRenamedHandler(gcbh);  OpenFcn=TD.InterfaceBlock.ModelCallbacks.OpenGUI( gcbh );  CloseFcn=TD.InterfaceBlock.ModelCallbacks.CloseGUI( gcbh );
      mask Display:
      | image('InterfaceBlock.png','center');
      | port_label('input',1, 'fromWheelSystem');
      | port_label('output',1, 'FrontLeft_Wheel_RotAcc[rad/s**2]');
      | port_label('output',2, 'FrontRight_Wheel_RotAcc[rad/s**2]');
      | port_label('output',3, 'RearLeft_Wheel_RotAcc[rad/s**2]');
      | port_label('output',4, 'RearRight_Wheel_RotAcc[rad/s**2]');
      | port_label('output',5, 'FrontLeft_Wheel_RotSpd[rad/s]');
      | port_label('output',6, 'FrontRight_Wheel_RotSpd[rad/s]');
      | port_label('output',7, 'RearLeft_Wheel_RotSpd[rad/s]');
      | port_label('output',8, 'RearRight_Wheel_RotSpd[rad/s]');
      | port_label('output',9, 'FrontLeft_Wheel_DriveBrakeTrq_wrt_WheelRotAxis(VehSys)[Nm]');
      | port_label('output',10, 'FrontRight_Wheel_DriveBrakeTrq_wrt_WheelRotAxis(VehSys)[Nm]');
      | port_label('output',11, 'RearLeft_Wheel_DriveBrakeTrq_wrt_WheelRotAxis(VehSys)[Nm]');
      | port_label('output',12, 'RearRight_Wheel_DriveBrakeTrq_wrt_WheelRotAxis(VehSys)[Nm]');
      | port_label('output',13, 'TotalResistanceTorque[Nm]');
      | port_label('output',14, 'FrontLeft_Wheel_RotAxisInrt[kg*m**2]');
      | port_label('output',15, 'FrontRight_Wheel_RotAxisInrt[kg*m**2]');
      | port_label('output',16, 'RearLeft_Wheel_RotAxisInrt[kg*m**2]');
      | port_label('output',17, 'RearRight_Wheel_RotAxisInrt[kg*m**2]');
      | port_label('output',18, 'VehBodyReplacementInrt[kg*m**2]');
      | port_label('output',19, 'KinematicWheelActiveFlag[0;1]');
  Memory : Memory  InheritSampleTime=on
  Memory1 : Memory  InheritSampleTime=on
  Memory2 : Memory  InheritSampleTime=on
  Terminator5 : Terminator
  Use IdleSpd if InitialEngineSpeed < 0 : Switch
  InitEngSpd[rad/s] : Outport  VectorParamsAs1DForOutWhenUnconnected=off
  InitialGear[-4;20] : Outport  Port=2  VectorParamsAs1DForOutWhenUnconnected=off
  IndicatedTrq[Nm] : Outport  Port=3  VectorParamsAs1DForOutWhenUnconnected=off
  EngFrictionTrq[Nm] : Outport  Port=4  VectorParamsAs1DForOutWhenUnconnected=off
  EngInrt[kg*m**2] : Outport  Port=5  VectorParamsAs1DForOutWhenUnconnected=off
  "DerivativeOfEngTrq_wrt_CrankAng[Nm/rad] " : Outport  Port=6  VectorParamsAs1DForOutWhenUnconnected=off
  "DerivativeOfEngTrq_wrt_EngSpd[Nm/(rad/s)] " : Outport  Port=7  VectorParamsAs1DForOutWhenUnconnected=off
  ClutchPos[0_1] : Outport  Port=8  VectorParamsAs1DForOutWhenUnconnected=off
  AutomatedManualClutchPos[0_1] : Outport  Port=9  VectorParamsAs1DForOutWhenUnconnected=off
  ManualGear[-4;20] : Outport  Port=10  VectorParamsAs1DForOutWhenUnconnected=off
  AutomaticGear[-4;20] : Outport  Port=11  VectorParamsAs1DForOutWhenUnconnected=off
  FrontLeftWheelRotSpd[rad/s] : Outport  Port=12  VectorParamsAs1DForOutWhenUnconnected=off
  FrontRightWheelRotSpd[rad/s] : Outport  Port=13  VectorParamsAs1DForOutWhenUnconnected=off
  FrontLeftWheelRotAcc[rad/s**2] : Outport  Port=14  VectorParamsAs1DForOutWhenUnconnected=off
  FrontRightWheelRotAcc[rad/s**2] : Outport  Port=15  VectorParamsAs1DForOutWhenUnconnected=off
  RearLeftWheelRotSpd[rad/s] : Outport  Port=16  VectorParamsAs1DForOutWhenUnconnected=off
  RearRightWheelRotSpd[rad/s] : Outport  Port=17  VectorParamsAs1DForOutWhenUnconnected=off
  RearLeftWheelRotAcc[rad/s**2] : Outport  Port=18  VectorParamsAs1DForOutWhenUnconnected=off
  RearRightWheelRotAcc[rad/s**2] : Outport  Port=19  VectorParamsAs1DForOutWhenUnconnected=off
  FrontLeftCircumferentialTrq[Nm] : Outport  Port=20  VectorParamsAs1DForOutWhenUnconnected=off
  FrontRightCircumferentialTrq[Nm] : Outport  Port=21  VectorParamsAs1DForOutWhenUnconnected=off
  RearLeftCircumferentialTrq[Nm] : Outport  Port=22  VectorParamsAs1DForOutWhenUnconnected=off
  RearRightCircumferentialTrq[Nm] : Outport  Port=23  VectorParamsAs1DForOutWhenUnconnected=off
  FrontLeftWheelRotAxisInrt[kg*m**2] : Outport  Port=24  VectorParamsAs1DForOutWhenUnconnected=off
  FrontRightWheelRotAxisInrt[kg*m**2] : Outport  Port=25  VectorParamsAs1DForOutWhenUnconnected=off
  RearLeftWheelRotAxisInrt[kg*m**2] : Outport  Port=26  VectorParamsAs1DForOutWhenUnconnected=off
  RearRightWheelRotAxisInrt[kg*m**2] : Outport  Port=27  VectorParamsAs1DForOutWhenUnconnected=off
  wires:
  InputFromEngine/6(EngIdleSpd[rad/s]___UNIQUE_1) -> Use IdleSpd if InitialEngineSpeed < 0/3
  fromDrivetrainControlUnit/1 -> InputFromDrivetrainControlUnit/1(fromDrivetrainControlUnit)
  InputFromDrivetrainControlUnit/2(AutomatedManualClutchPos[0_1]___UNIQUE_1) -> Memory1/1
  InputFromDrivetrainControlUnit/1(AutomaticGear[-4;20]___UNIQUE_1) -> Memory2/1
  InputFromCTRL/4(ManualGear[-4;20]___UNIQUE_1) -> Memory/1
  Add1/1 -> IndicatedTrq[Nm]/1
  fromAuxiliaries/1 -> InputFromAuxiliaries/1(fromAuxiliaries)
  fromEngine/1 -> InputFromEngine/1(fromEngine)
  Add2/1 -> EngInrt[kg*m**2]/1
  InputFromEngine/1(EngInrt[kg*m**2]___UNIQUE_1) -> Add2/1
  InputFromAuxiliaries/1(StarterInrt[kgm**2]___UNIQUE_1) -> Add2/2
  InputFromAuxiliaries/2(StarterTrq[Nm]___UNIQUE_1) -> Add1/2
  InputFromEngine/3(DerivativeOfEngTrq_wrt_CrankAng[Nm/rad]___UNIQUE_1) -> "DerivativeOfEngTrq_wrt_CrankAng[Nm/rad] "/1
  InputFromEngine/4(DerivativeOfEngTrq_wrt_EngSpd[Nm/(rad/s)]___UNIQUE_1) -> "DerivativeOfEngTrq_wrt_EngSpd[Nm/(rad/s)] "/1
  InputFromEngine/5(MeanEngFrictionTrq[Nm]___UNIQUE_1) -> EngFrictionTrq[Nm]/1, Add3/2
  InputFromEngine/2(EngTrq[Nm]___UNIQUE_1) -> Add3/1
  Add3/1 -> Add1/1
  fromCTRL/1 -> InputFromCTRL/1(fromCTRL)
  fromWheelSystem/1 -> InputFromWheelSystem/1(fromWheelSystem)
  fromElectricalSystem/1 -> Terminator5/1
  InputFromWheelSystem/1(FrontLeft_Wheel_RotAcc[rad/s**2]___UNIQUE_1) -> FrontLeftWheelRotAcc[rad/s**2]/1
  InputFromWheelSystem/2(FrontRight_Wheel_RotAcc[rad/s**2]___UNIQUE_1) -> FrontRightWheelRotAcc[rad/s**2]/1
  InputFromWheelSystem/3(RearLeft_Wheel_RotAcc[rad/s**2]___UNIQUE_1) -> RearLeftWheelRotAcc[rad/s**2]/1
  InputFromWheelSystem/4(RearRight_Wheel_RotAcc[rad/s**2]___UNIQUE_1) -> RearRightWheelRotAcc[rad/s**2]/1
  InputFromWheelSystem/5(FrontLeft_Wheel_RotSpd[rad/s]___UNIQUE_1) -> FrontLeftWheelRotSpd[rad/s]/1
  InputFromWheelSystem/6(FrontRight_Wheel_RotSpd[rad/s]___UNIQUE_1) -> FrontRightWheelRotSpd[rad/s]/1
  InputFromWheelSystem/7(RearLeft_Wheel_RotSpd[rad/s]___UNIQUE_1) -> RearLeftWheelRotSpd[rad/s]/1
  InputFromWheelSystem/8(RearRight_Wheel_RotSpd[rad/s]___UNIQUE_1) -> RearRightWheelRotSpd[rad/s]/1
  InputFromWheelSystem/9(FrontLeft_Wheel_DriveBrakeTrq_wrt_WheelRotAxis(VehSys)[Nm]___UNIQUE_1) -> Determine Torques and Inertias based on Wheel System Type/1
  InputFromWheelSystem/10(FrontRight_Wheel_DriveBrakeTrq_wrt_WheelRotAxis(VehSys)[Nm]___UNIQUE_1) -> Determine Torques and Inertias based on Wheel System Type/2
  InputFromWheelSystem/11(RearLeft_Wheel_DriveBrakeTrq_wrt_WheelRotAxis(VehSys)[Nm]___UNIQUE_1) -> Determine Torques and Inertias based on Wheel System Type/3
  InputFromWheelSystem/12(RearRight_Wheel_DriveBrakeTrq_wrt_WheelRotAxis(VehSys)[Nm]___UNIQUE_1) -> Determine Torques and Inertias based on Wheel System Type/4
  InputFromWheelSystem/13(TotalResistanceTorque[Nm]___UNIQUE_1) -> Determine Torques and Inertias based on Wheel System Type/5
  InputFromWheelSystem/14(FrontLeft_Wheel_RotAxisInrt[kg*m**2]___UNIQUE_1) -> Determine Torques and Inertias based on Wheel System Type/6
  InputFromWheelSystem/15(FrontRight_Wheel_RotAxisInrt[kg*m**2]___UNIQUE_1) -> Determine Torques and Inertias based on Wheel System Type/7
  InputFromWheelSystem/16(RearLeft_Wheel_RotAxisInrt[kg*m**2]___UNIQUE_1) -> Determine Torques and Inertias based on Wheel System Type/8
  InputFromWheelSystem/17(RearRight_Wheel_RotAxisInrt[kg*m**2]___UNIQUE_1) -> Determine Torques and Inertias based on Wheel System Type/9
  InputFromWheelSystem/18(VehBodyReplacementInrt[kg*m**2]___UNIQUE_1) -> Determine Torques and Inertias based on Wheel System Type/10
  InputFromWheelSystem/19(KinematicWheelActiveFlag[0;1]___UNIQUE_1) -> Determine Torques and Inertias based on Wheel System Type/11
  DrivetrainInfo/1 -> Determine Torques and Inertias based on Wheel System Type/12
  Demux2/1 -> FrontLeftWheelRotAxisInrt[kg*m**2]/1
  Demux2/2 -> FrontRightWheelRotAxisInrt[kg*m**2]/1
  Determine Torques and Inertias based on Wheel System Type/3 -> Demux2/1
  Demux1/1 -> RearLeftCircumferentialTrq[Nm]/1
  Demux1/2 -> RearRightCircumferentialTrq[Nm]/1
  Determine Torques and Inertias based on Wheel System Type/2 -> Demux1/1
  Demux4/1 -> FrontLeftCircumferentialTrq[Nm]/1
  Demux4/2 -> FrontRightCircumferentialTrq[Nm]/1
  Determine Torques and Inertias based on Wheel System Type/1 -> Demux4/1
  Demux5/1 -> RearLeftWheelRotAxisInrt[kg*m**2]/1
  Demux5/2 -> RearRightWheelRotAxisInrt[kg*m**2]/1
  Determine Torques and Inertias based on Wheel System Type/4 -> Demux5/1
  InputFromCTRL/3(ClutchPos[0_1]___UNIQUE_1) -> ClutchPos[0_1]/1
  Memory1/1 -> AutomatedManualClutchPos[0_1]/1
  Memory/1 -> ManualGear[-4;20]/1
  Memory2/1 -> AutomaticGear[-4;20]/1
  InputFromCTRL/2(InitialGear[-4;20]___UNIQUE_1) -> InitialGear[-4;20]/1
  Use IdleSpd if InitialEngineSpeed < 0/1 -> InitEngSpd[rad/s]/1
  InputFromCTRL/1(InitialEngineSpeed[rad/s]___UNIQUE_1) -> Use IdleSpd if InitialEngineSpeed < 0/1, Use IdleSpd if InitialEngineSpeed < 0/2
